simulink model "MagLev_1DOF_Slice_with_noise"  (R2020b)
settings: Solver=ode45  StartTime=0.0  StopTime=15  FixedStep=1e-5  RelTol=1e-3
values from neighbouring files (symbols this model uses):
  c = 0.005    [setup.m]
  caseNumber = 2    [setup.m]
  chi_0 = 0    [setup.m]
  dY_0 = 0.5    [setup.m]
  epsilon = 1e-3    (= 0.001)    [setup.m]
  eth10 = 0.0001    [setup.m]
  g = 9.81    [setup.m]
  gamma_ALCOS = 1000    [setup.m]
  gamma_s = 10    [setup.m]
  gamma_SLICE = 100    [setup.m]
  gamma_y = 10    [setup.m]
  k = 1    [setup.m]
  k0 = kk^3    (= 1000)    [setup.m]
  k1 = 3*kk^2    (= 300)    [setup.m]
  k2 = 3*kk    (= 30)    [setup.m]
  lambda_0 = -0.02    [setup.m]
  m = 0.0844    [setup.m]
  mu = 10    [setup.m]
  nu = 1    [setup.m]
  Omega = [ ... (first row only)    [setup.m]
  R = 2.52    [setup.m]
  s = [1; 2; 10; 20; 5; 7]    [setup.m]
  tt1 = 1    [setup.m]
  tt2 = 3    [setup.m]
  tt3 = 5    [setup.m]
  tt4 = 7    [setup.m]
  Y_0 = -1    [setup.m]
(part 2 of 2)

== matlab function MagLev_1DOF_Slice_with_noise/regression model/  regression model/terms of the real q4 ==
  data: q1 input; q2 input; phi1 input; phi2 input; psi input; omega1 input; omega2 input; W1 input size=10; W2 input size=6; W3 input size=2; k parameter; g parameter; m parameter; z output size=1; phi output size=6; w1 output size=10; w2 output size=6; lambda_0 parameter; w3 output; mu parameter
function [z, phi, w1, w2, w3] = fcn( q1, q2, phi1, phi2, psi, omega1, omega2, W1, W2, W3, k, g, m, lambda_0, mu)

theta = lambda_0;

psi1 = psi;
psi2 = psi1^2;

w1psi1 = W1(1);
w1psi2 = W1(2);
w1psi1w1psi1 = W1(3);
w1psi1w1psi2 = W1(4);
w1psi1w2psi1 = W1(5);
w1psi1w2psi2 = W1(6);
w1a1w1psi1 = W1(7);
w1a1w1psi2 = W1(8);
w1a1w2psi1 = W1(9);
w1a1w2psi2 = W1(10);

w2psi1 = W2(1);
w2psi2 = W2(2);
w2psi1w1psi1 = W2(3);
w2psi1w1psi2 = W2(4);
w2a1w1psi1 = W2(5);
w2a1w1psi2 = W2(6);

w3psi1 = W3(1);
w3psi2 = W3(2);

a1 = psi2 - 2*m*g*k;
psi1w1psi1 = psi1*w1psi1;
psi1w1psi2 = psi1*w1psi2;
psi1w2psi1 = psi1*w2psi1;
psi1w2psi2 = psi1*w2psi2;
a1w1psi1 = a1*w1psi1;
a1w1psi2 = a1*w1psi2;
a1w2psi1 = a1*w2psi1;
a1w2psi2 = a1*w2psi2;

w1 = [
  psi1;
  psi2;
  psi1w1psi1;
  psi1w1psi2;
  psi1w2psi1;
  psi1w2psi2;
  a1w1psi1;
  a1w1psi2;
  a1w2psi1;
  a1w2psi2
];

w2 = [
  psi1;
  psi2;
  psi1w1psi1;
  psi1w1psi2;
  a1w1psi1;
  a1w1psi2
];

w3 = [
  psi1;
  psi2;
];

% z = 2*k*mu*(k*m*q1*phi2 - q2*phi1) ...
%     + w2psi2*w1a1w1psi2 ...
%     - w1psi2*w1a1w2psi2 ...
%     - w1psi2*w2a1w1psi2;
% 
% phi1 =  ( omega1*w2psi2 - omega2*w1psi2 )*2*k^2*m*mu ...
%     - ( 2*w2psi1*w1a1w1psi2 + w2psi2*(2*w1psi1w1psi2 + 2*w1a1w1psi1) ) ...
%     + ( 2*w1psi1*w1a1w2psi2 + w1psi2*(2*w1psi1w2psi2 + 2*w1a1w2psi1) ) ...
%     + (2*w1psi1*w2a1w1psi2 + w1psi2*(2*w2psi1w1psi2 + 2*w2a1w1psi1));
%     
% phi2 = ( omega1*w2psi1 - omega2*w1psi1 )*4*k^2*m*mu ...
%     - ( w1a1w1psi2 + 4*w2psi1*(w1psi1w1psi2 + w1a1w1psi1) + w2psi2*(w1psi2 - 2*m*g*k + w2psi2 + 4*w1psi1w1psi1) ) ...
%     + ( w1a1w2psi2 + 4*w1psi1*(w1psi1w2psi2 + w1a1w2psi1) + w1psi2*(w1psi2 - 2*m*g*k + w3psi2 + 4*w1psi1w2psi1) ) ...
%     + (w2a1w1psi2 + 4*w1psi1*(w2psi1w1psi2 + w2a1w1psi1) + w1psi2*(w2psi2 - 2*m*g*k + w3psi2 + 4*w2psi1w1psi1));
% 
% phi3 = ( omega1 - omega2 )*2*k^2*m*mu ...
%     - ( 2*w1psi1w1psi2 + 2*w1a1w1psi1 + 2*w2psi1*(w1psi2 - 2*m*g*k + w2psi2 + 4*w1psi1w1psi1) + 2*w2psi2*(w1psi1 + w2psi1) ) ...
%     + ( 2*w1psi1w2psi2 + 2*w1a1w2psi1 + 2*w1psi1*(w1psi2 - 2*m*g*k + w3psi2 + 4*w1psi1w2psi1) + 2*w1psi2*(w1psi1 + w3psi1) ) ...
%     + (2*w2psi1w1psi2 + 2*w2a1w1psi1 + 2*w1psi1*(w2psi2 - 2*m*g*k + w3psi2 + 4*w2psi1w1psi1) + 2*w1psi2*(w2psi1 + w3psi1));
% 
% phi4 = - ( w1psi2 - 2*m*g*k + w2psi2 + 4*w1psi1w1psi1 + 4*w2psi1*(w1psi1 + w2psi1) + w2psi2 ) ...
%     + ( w1psi2 - 2*m*g*k + w3psi2 + 4*w1psi1w2psi1 + 4*w1psi1*(w1psi1 + w3psi1) + w1psi2 ) ...
%     + (w2psi2 - 2*m*g*k + w3psi2 + 4*w2psi1w1psi1 + 4*w1psi1*(w2psi1 + w3psi1) + w1psi2);

z = 2*k*mu*(k*m*q1*phi2 - q2*phi1) ...
    - w1psi2*(w1a1w2psi2 + w2a1w1psi2) ...
    + w2psi2*w1a1w1psi2;

phi1 =  ( omega1*w2psi2 - omega2*w1psi2 )*2*k^2*m*mu ...
    + 2*w1psi1*(w1a1w2psi2 + w2a1w1psi2) ...
    + 2*w1psi2*(w1psi1w2psi2 + w1a1w2psi1 + w2psi1w1psi2 + w2a1w1psi1) ...
    - 2*w2psi1*w1a1w1psi2 ...
    - 2*w2psi2*(w1psi1w1psi2 + w1a1w1psi1);
    
phi2 = ( omega1*w2psi1 - omega2*w1psi1 )*4*k^2*m*mu ...
    + 2*m*g*k*(w2psi2 - 2*w1psi2) ...
    + (w1psi2)^2 - (w2psi2)^2 ...
    + 4*w1psi1*(w1psi1w2psi2 + w1a1w2psi1 + w2psi1w1psi2 + w2a1w1psi1) ...
    + 2*w1psi2*(w3psi2 + 2*w1psi1w2psi1 + 2*w2psi1w1psi1) ...
    - 4*w2psi1*(w1psi1w1psi2 + w1a1w1psi1) ...
    - w1a1w1psi2 + w1a1w2psi2 ...
    + w2a1w1psi2 ...
    - 4*w2psi2*w1psi1w1psi1;

phi3 = ( omega1 - omega2 )*2*k^2*m*mu ...
    + 4*m*g*k*(w2psi1 - 2*w1psi1)  ...
    + 4*w1psi1*(w1psi2 + w3psi2 + 2*w1psi1w2psi1 + 2*w2psi1w1psi1) ...
    + 4*w1psi2*w3psi1 ...
    - 4*w2psi1*( w2psi2 + 2*w1psi1w1psi1) ...
    - 2*w1psi1w1psi2 + 2*w1psi1w2psi2+ 2*w2psi1w1psi2 ...
    - 2*w1a1w1psi1+ 2*w1a1w2psi1 + 2*w2a1w1psi1;

phi4 = - 2*m*g*k + 2*w1psi2 - w2psi2 + 2*w3psi2 - 4*w2psi1*w2psi1 ...
    + 4*w1psi1*w1psi1 + 8*w1psi1*w3psi1 ...
    - 4*w1psi1w1psi1 + 4*w1psi1w2psi1 ...
    + 4*w2psi1w1psi1;

phi5 = - 2*w2psi1 + 4*w3psi1 + 4*w1psi1;

phi6 = 1;

phi = [
    phi1;
    phi2;
    phi3;
    phi4;
    phi5;
    phi6
];

== matlab function MagLev_1DOF_Slice_with_noise/Controller ==
  data: Yd input size=4; u output size=1; X input size=3; c parameter; k parameter; R parameter; g parameter; m parameter; k0 parameter; k1 parameter; k2 parameter
function u = fcn(Yd, X, c, k, R, g, m, k0, k1, k2)

Y = X(1);
dY = X(2)/m;
lambda = X(3);

F = 0.5*lambda^2/k;

v = Yd(4) - k2*( (F/m - g) - Yd(3) ) - k1*( dY - Yd(2) ) - k0*( Y - Yd(1));

u = sqrt(0.5*k/F)*m*v + R*(c - Y)*sqrt(2*F/k);

== matlab function MagLev_1DOF_Slice_with_noise/Controller1 ==
  data: Yd input size=4; u output size=1; X input size=3; c parameter; k parameter; R parameter; g parameter; m parameter; k0 parameter; k1 parameter; k2 parameter
function u = fcn(Yd, X, c, k, R, g, m, k0, k1, k2)

Y = X(1);
dY = X(2)/m;
lambda = X(3);

F = 0.5*lambda^2/k;

v = Yd(4) - k2*( (F/m - g) - Yd(3) ) - k1*( dY - Yd(2) ) - k0*( Y - Yd(1));

u = sqrt(0.5*k/F)*m*v + R*(c - Y)*sqrt(2*F/k);

== matlab function MagLev_1DOF_Slice_with_noise/regression model/Vectorize/q1/terms of the q1 est ==
  data: y input; u input; psi input; omega1 input; R parameter; term1 output; term2 output; term3 output
function [term1, term2, term3] = fcn( y, u, psi, omega1, R )

term1 = y*(u - R*y);
term2 = psi*omega1;
term3 = (u - R*y)*omega1;

== matlab function MagLev_1DOF_Slice_with_noise/Estimation ALCOS/DREM2 ==
  data: in1 input size=6; newreg output; in2 input size=6 =in2; y1 output; y2 output; y3 output; y4 output; in3 input size=6; in4 input size=6; in5 input size=6; y5 output
function [newreg,y1,y2,y3,y4,y5] = fcn(in1,in2,in3,in4,in5)


a11=in1(1); a12=in1(2); a13=in1(3); a14=in1(4); a15=in1(5);

a21=in2(1); a22=in2(2); a23=in2(3); a24=in2(4); a25=in2(5);

a31=in3(1); a32=in3(2); a33=in3(3); a34=in3(4); a35=in3(5);

a41=in4(1); a42=in4(2); a43=in4(3); a44=in4(4); a45=in4(5);

a51=in5(1); a52=in5(2); a53=in5(3); a54=in5(4); a55=in5(5);

RegM=[a11  a12  a13  a14  a15; a21  a22  a23  a24  a25; a31  a32  a33  a34  a35; a41  a42  a43  a44  a45; a51  a52  a53  a54  a55];

newreg=det(RegM);

adj1=[a22*a33*a44*a55 - a22*a33*a45*a54 - a22*a34*a43*a55 + a22*a34*a45*a53 + a22*a35*a43*a54 - a22*a35*a44*a53 - a23*a32*a44*a55 + a23*a32*a45*a54 ...
+ a23*a34*a42*a55 - a23*a34*a45*a52 - a23*a35*a42*a54 + a23*a35*a44*a52 + a24*a32*a43*a55 - a24*a32*a45*a53 - a24*a33*a42*a55 + a24*a33*a45*a52 ...
+ a24*a35*a42*a53 - a24*a35*a43*a52 - a25*a32*a43*a54 + a25*a32*a44*a53 + a25*a33*a42*a54 - a25*a33*a44*a52 - a25*a34*a42*a53 + a25*a34*a43*a52, 
a12*a33*a45*a54 - a12*a33*a44*a55 + a12*a34*a43*a55 - a12*a34*a45*a53 - a12*a35*a43*a54 + a12*a35*a44*a53 + a13*a32*a44*a55 - a13*a32*a45*a54 - ...
a13*a34*a42*a55 + a13*a34*a45*a52 + a13*a35*a42*a54 - a13*a35*a44*a52 - a14*a32*a43*a55 + a14*a32*a45*a53 + a14*a33*a42*a55 - a14*a33*a45*a52 - ...
a14*a35*a42*a53 + a14*a35*a43*a52 + a15*a32*a43*a54 - a15*a32*a44*a53 - a15*a33*a42*a54 + a15*a33*a44*a52 + a15*a34*a42*a53 - a15*a34*a43*a52, 
a12*a23*a44*a55 - a12*a23*a45*a54 - a12*a24*a43*a55 + a12*a24*a45*a53 + a12*a25*a43*a54 - a12*a25*a44*a53 - a13*a22*a44*a55 + a13*a22*a45*a54 ...
+ a13*a24*a42*a55 - a13*a24*a45*a52 - a13*a25*a42*a54 + a13*a25*a44*a52 + a14*a22*a43*a55 - a14*a22*a45*a53 - a14*a23*a42*a55 + a14*a23*a45*a52 ...
+ a14*a25*a42*a53 - a14*a25*a43*a52 - a15*a22*a43*a54 + a15*a22*a44*a53 + a15*a23*a42*a54 - a15*a23*a44*a52 - a15*a24*a42*a53 + a15*a24*a43*a52, 
a12*a23*a35*a54 - a12*a23*a34*a55 + a12*a24*a33*a55 - a12*a24*a35*a53 - a12*a25*a33*a54 + a12*a25*a34*a53 + a13*a22*a34*a55 - a13*a22*a35*a54 ...
- a13*a24*a32*a55 + a13*a24*a35*a52 + a13*a25*a32*a54 - a13*a25*a34*a52 - a14*a22*a33*a55 + a14*a22*a35*a53 + a14*a23*a32*a55 - a14*a23*a35*a52 ...
- a14*a25*a32*a53 + a14*a25*a33*a52 + a15*a22*a33*a54 - a15*a22*a34*a53 - a15*a23*a32*a54 + a15*a23*a34*a52 + a15*a24*a32*a53 - a15*a24*a33*a52, 
a12*a23*a34*a45 - a12*a23*a35*a44 - a12*a24*a33*a45 + a12*a24*a35*a43 + a12*a25*a33*a44 - a12*a25*a34*a43 - a13*a22*a34*a45 + a13*a22*a35*a44 ...
+ a13*a24*a32*a45 - a13*a24*a35*a42 - a13*a25*a32*a44 + a13*a25*a34*a42 + a14*a22*a33*a45 - a14*a22*a35*a43 - a14*a23*a32*a45 + a14*a23*a35*a42 ...
+ a14*a25*a32*a43 - a14*a25*a33*a42 - a15*a22*a33*a44 + a15*a22*a34*a43 + a15*a23*a32*a44 - a15*a23*a34*a42 - a15*a24*a32*a43 + a15*a24*a33*a42];

adj2=[a21*a33*a45*a54 - a21*a33*a44*a55 + a21*a34*a43*a55 - a21*a34*a45*a53 - a21*a35*a43*a54 + a21*a35*a44*a53 + a23*a31*a44*a55 - a23*a31*a45*a54 ...
- a23*a34*a41*a55 + a23*a34*a45*a51 + a23*a35*a41*a54 - a23*a35*a44*a51 - a24*a31*a43*a55 + a24*a31*a45*a53 + a24*a33*a41*a55 - a24*a33*a45*a51 ...
- a24*a35*a41*a53 + a24*a35*a43*a51 + a25*a31*a43*a54 - a25*a31*a44*a53 - a25*a33*a41*a54 + a25*a33*a44*a51 + a25*a34*a41*a53 - a25*a34*a43*a51, 
a11*a33*a44*a55 - a11*a33*a45*a54 - a11*a34*a43*a55 + a11*a34*a45*a53 + a11*a35*a43*a54 - a11*a35*a44*a53 - a13*a31*a44*a55 + a13*a31*a45*a54 ...
+ a13*a34*a41*a55 - a13*a34*a45*a51 - a13*a35*a41*a54 + a13*a35*a44*a51 + a14*a31*a43*a55 - a14*a31*a45*a53 - a14*a33*a41*a55 + a14*a33*a45*a51 ...
+ a14*a35*a41*a53 - a14*a35*a43*a51 - a15*a31*a43*a54 + a15*a31*a44*a53 + a15*a33*a41*a54 - a15*a33*a44*a51 - a15*a34*a41*a53 + a15*a34*a43*a51, 
a11*a23*a45*a54 - a11*a23*a44*a55 + a11*a24*a43*a55 - a11*a24*a45*a53 - a11*a25*a43*a54 + a11*a25*a44*a53 + a13*a21*a44*a55 - a13*a21*a45*a54 ...
- a13*a24*a41*a55 + a13*a24*a45*a51 + a13*a25*a41*a54 - a13*a25*a44*a51 - a14*a21*a43*a55 + a14*a21*a45*a53 + a14*a23*a41*a55 - a14*a23*a45*a51...
- a14*a25*a41*a53 + a14*a25*a43*a51 + a15*a21*a43*a54 - a15*a21*a44*a53 - a15*a23*a41*a54 + a15*a23*a44*a51 + a15*a24*a41*a53 - a15*a24*a43*a51, 
a11*a23*a34*a55 - a11*a23*a35*a54 - a11*a24*a33*a55 + a11*a24*a35*a53 + a11*a25*a33*a54 - a11*a25*a34*a53 - a13*a21*a34*a55 + a13*a21*a35*a54 ...
+ a13*a24*a31*a55 - a13*a24*a35*a51 - a13*a25*a31*a54 + a13*a25*a34*a51 + a14*a21*a33*a55 - a14*a21*a35*a53 - a14*a23*a31*a55 + a14*a23*a35*a51 ...
+ a14*a25*a31*a53 - a14*a25*a33*a51 - a15*a21*a33*a54 + a15*a21*a34*a53 + a15*a23*a31*a54 - a15*a23*a34*a51 - a15*a24*a31*a53 + a15*a24*a33*a51, 
a11*a23*a35*a44 - a11*a23*a34*a45 + a11*a24*a33*a45 - a11*a24*a35*a43 - a11*a25*a33*a44 + a11*a25*a34*a43 + a13*a21*a34*a45 - a13*a21*a35*a44...
- a13*a24*a31*a45 + a13*a24*a35*a41 + a13*a25*a31*a44 - a13*a25*a34*a41 - a14*a21*a33*a45 + a14*a21*a35*a43 + a14*a23*a31*a45 - a14*a23*a35*a41 ...
- a14*a25*a31*a43 + a14*a25*a33*a41 + a15*a21*a33*a44 - a15*a21*a34*a43 - a15*a23*a31*a44 + a15*a23*a34*a41 + a15*a24*a31*a43 - a15*a24*a33*a41];

adj3=[a21*a32*a44*a55 - a21*a32*a45*a54 - a21*a34*a42*a55 + a21*a34*a45*a52 + a21*a35*a42*a54 - a21*a35*a44*a52 - a22*a31*a44*a55 + a22*a31*a45*a54 ...
+ a22*a34*a41*a55 - a22*a34*a45*a51 - a22*a35*a41*a54 + a22*a35*a44*a51 + a24*a31*a42*a55 - a24*a31*a45*a52 - a24*a32*a41*a55 + a24*a32*a45*a51...
+ a24*a35*a41*a52 - a24*a35*a42*a51 - a25*a31*a42*a54 + a25*a31*a44*a52 + a25*a32*a41*a54 - a25*a32*a44*a51 - a25*a34*a41*a52 + a25*a34*a42*a51, 
a11*a32*a45*a54 - a11*a32*a44*a55 + a11*a34*a42*a55 - a11*a34*a45*a52 - a11*a35*a42*a54 + a11*a35*a44*a52 + a12*a31*a44*a55 - a12*a31*a45*a54 ...
- a12*a34*a41*a55 + a12*a34*a45*a51 + a12*a35*a41*a54 - a12*a35*a44*a51 - a14*a31*a42*a55 + a14*a31*a45*a52 + a14*a32*a41*a55 - a14*a32*a45*a51 ...
- a14*a35*a41*a52 + a14*a35*a42*a51 + a15*a31*a42*a54 - a15*a31*a44*a52 - a15*a32*a41*a54 + a15*a32*a44*a51 + a15*a34*a41*a52 - a15*a34*a42*a51, 
a11*a22*a44*a55 - a11*a22*a45*a54 - a11*a24*a42*a55 + a11*a24*a45*a52 + a11*a25*a42*a54 - a11*a25*a44*a52 - a12*a21*a44*a55 + a12*a21*a45*a54 ...
+ a12*a24*a41*a55 - a12*a24*a45*a51 - a12*a25*a41*a54 + a12*a25*a44*a51 + a14*a21*a42*a55 - a14*a21*a45*a52 - a14*a22*a41*a55 + a14*a22*a45*a51 ...
+ a14*a25*a41*a52 - a14*a25*a42*a51 - a15*a21*a42*a54 + a15*a21*a44*a52 + a15*a22*a41*a54 - a15*a22*a44*a51 - a15*a24*a41*a52 + a15*a24*a42*a51, 
a11*a22*a35*a54 - a11*a22*a34*a55 + a11*a24*a32*a55 - a11*a24*a35*a52 - a11*a25*a32*a54 + a11*a25*a34*a52 + a12*a21*a34*a55 - a12*a21*a35*a54...
- a12*a24*a31*a55 + a12*a24*a35*a51 + a12*a25*a31*a54 - a12*a25*a34*a51 - a14*a21*a32*a55 + a14*a21*a35*a52 + a14*a22*a31*a55 - a14*a22*a35*a51 ...
- a14*a25*a31*a52 + a14*a25*a32*a51 + a15*a21*a32*a54 - a15*a21*a34*a52 - a15*a22*a31*a54 + a15*a22*a34*a51 + a15*a24*a31*a52 - a15*a24*a32*a51, 
a11*a22*a34*a45 - a11*a22*a35*a44 - a11*a24*a32*a45 + a11*a24*a35*a42 + a11*a25*a32*a44 - a11*a25*a34*a42 - a12*a21*a34*a45 + a12*a21*a35*a44 ...
+ a12*a24*a31*a45 - a12*a24*a35*a41 - a12*a25*a31*a44 + a12*a25*a34*a41 + a14*a21*a32*a45 - a14*a21*a35*a42 - a14*a22*a31*a45 + a14*a22*a35*a41 ...
+ a14*a25*a31*a42 - a14*a25*a32*a41 - a15*a21*a32*a44 + a15*a21*a34*a42 + a15*a22*a31*a44 - a15*a22*a34*a41 - a15*a24*a31*a42 + a15*a24*a32*a41];

adj4=[a21*a32*a45*a53 - a21*a32*a43*a55 + a21*a33*a42*a55 - a21*a33*a45*a52 - a21*a35*a42*a53 + a21*a35*a43*a52 + a22*a31*a43*a55 - a22*a31*a45*a53 ...
- a22*a33*a41*a55 + a22*a33*a45*a51 + a22*a35*a41*a53 - a22*a35*a43*a51 - a23*a31*a42*a55 + a23*a31*a45*a52 + a23*a32*a41*a55 - a23*a32*a45*a51 ...
- a23*a35*a41*a52 + a23*a35*a42*a51 + a25*a31*a42*a53 - a25*a31*a43*a52 - a25*a32*a41*a53 + a25*a32*a43*a51 + a25*a33*a41*a52 - a25*a33*a42*a51, 
a11*a32*a43*a55 - a11*a32*a45*a53 - a11*a33*a42*a55 + a11*a33*a45*a52 + a11*a35*a42*a53 - a11*a35*a43*a52 - a12*a31*a43*a55 + a12*a31*a45*a53 ...
+ a12*a33*a41*a55 - a12*a33*a45*a51 - a12*a35*a41*a53 + a12*a35*a43*a51 + a13*a31*a42*a55 - a13*a31*a45*a52 - a13*a32*a41*a55 + a13*a32*a45*a51 ...
+ a13*a35*a41*a52 - a13*a35*a42*a51 - a15*a31*a42*a53 + a15*a31*a43*a52 + a15*a32*a41*a53 - a15*a32*a43*a51 - a15*a33*a41*a52 + a15*a33*a42*a51, 
a11*a22*a45*a53 - a11*a22*a43*a55 + a11*a23*a42*a55 - a11*a23*a45*a52 - a11*a25*a42*a53 + a11*a25*a43*a52 + a12*a21*a43*a55 - a12*a21*a45*a53 ...
- a12*a23*a41*a55 + a12*a23*a45*a51 + a12*a25*a41*a53 - a12*a25*a43*a51 - a13*a21*a42*a55 + a13*a21*a45*a52 + a13*a22*a41*a55 - a13*a22*a45*a51...
- a13*a25*a41*a52 + a13*a25*a42*a51 + a15*a21*a42*a53 - a15*a21*a43*a52 - a15*a22*a41*a53 + a15*a22*a43*a51 + a15*a23*a41*a52 - a15*a23*a42*a51, 
a11*a22*a33*a55 - a11*a22*a35*a53 - a11*a23*a32*a55 + a11*a23*a35*a52 + a11*a25*a32*a53 - a11*a25*a33*a52 - a12*a21*a33*a55 + a12*a21*a35*a53 ...
+ a12*a23*a31*a55 - a12*a23*a35*a51 - a12*a25*a31*a53 + a12*a25*a33*a51 + a13*a21*a32*a55 - a13*a21*a35*a52 - a13*a22*a31*a55 + a13*a22*a35*a51 ...
+ a13*a25*a31*a52 - a13*a25*a32*a51 - a15*a21*a32*a53 + a15*a21*a33*a52 + a15*a22*a31*a53 - a15*a22*a33*a51 - a15*a23*a31*a52 + a15*a23*a32*a51,
a11*a22*a35*a43 - a11*a22*a33*a45 + a11*a23*a32*a45 - a11*a23*a35*a42 - a11*a25*a32*a43 + a11*a25*a33*a42 + a12*a21*a33*a45 - a12*a21*a35*a43 ...
- a12*a23*a31*a45 + a12*a23*a35*a41 + a12*a25*a31*a43 - a12*a25*a33*a41 - a13*a21*a32*a45 + a13*a21*a35*a42 + a13*a22*a31*a45 - a13*a22*a35*a41 ...
- a13*a25*a31*a42 + a13*a25*a32*a41 + a15*a21*a32*a43 - a15*a21*a33*a42 - a15*a22*a31*a43 + a15*a22*a33*a41 + a15*a23*a31*a42 - a15*a23*a32*a41];

adj5=[a21*a32*a43*a54 - a21*a32*a44*a53 - a21*a33*a42*a54 + a21*a33*a44*a52 + a21*a34*a42*a53 - a21*a34*a43*a52 - a22*a31*a43*a54 + a22*a31*a44*a53...
+ a22*a33*a41*a54 - a22*a33*a44*a51 - a22*a34*a41*a53 + a22*a34*a43*a51 + a23*a31*a42*a54 - a23*a31*a44*a52 - a23*a32*a41*a54 + a23*a32*a44*a51 ...
+ a23*a34*a41*a52 - a23*a34*a42*a51 - a24*a31*a42*a53 + a24*a31*a43*a52 + a24*a32*a41*a53 - a24*a32*a43*a51 - a24*a33*a41*a52 + a24*a33*a42*a51, 
a11*a32*a44*a53 - a11*a32*a43*a54 + a11*a33*a42*a54 - a11*a33*a44*a52 - a11*a34*a42*a53 + a11*a34*a43*a52 + a12*a31*a43*a54 - a12*a31*a44*a53 ...
- a12*a33*a41*a54 + a12*a33*a44*a51 + a12*a34*a41*a53 - a12*a34*a43*a51 - a13*a31*a42*a54 + a13*a31*a44*a52 + a13*a32*a41*a54 - a13*a32*a44*a51 ...
- a13*a34*a41*a52 + a13*a34*a42*a51 + a14*a31*a42*a53 - a14*a31*a43*a52 - a14*a32*a41*a53 + a14*a32*a43*a51 + a14*a33*a41*a52 - a14*a33*a42*a51,
a11*a22*a43*a54 - a11*a22*a44*a53 - a11*a23*a42*a54 + a11*a23*a44*a52 + a11*a24*a42*a53 - a11*a24*a43*a52 - a12*a21*a43*a54 + a12*a21*a44*a53 ...
+ a12*a23*a41*a54 - a12*a23*a44*a51 - a12*a24*a41*a53 + a12*a24*a43*a51 + a13*a21*a42*a54 - a13*a21*a44*a52 - a13*a22*a41*a54 + a13*a22*a44*a51...
+ a13*a24*a41*a52 - a13*a24*a42*a51 - a14*a21*a42*a53 + a14*a21*a43*a52 + a14*a22*a41*a53 - a14*a22*a43*a51 - a14*a23*a41*a52 + a14*a23*a42*a51,
a11*a22*a34*a53 - a11*a22*a33*a54 + a11*a23*a32*a54 - a11*a23*a34*a52 - a11*a24*a32*a53 + a11*a24*a33*a52 + a12*a21*a33*a54 - a12*a21*a34*a53 ...
- a12*a23*a31*a54 + a12*a23*a34*a51 + a12*a24*a31*a53 - a12*a24*a33*a51 - a13*a21*a32*a54 + a13*a21*a34*a52 + a13*a22*a31*a54 - a13*a22*a34*a51 ...
- a13*a24*a31*a52 + a13*a24*a32*a51 + a14*a21*a32*a53 - a14*a21*a33*a52 - a14*a22*a31*a53 + a14*a22*a33*a51 + a14*a23*a31*a52 - a14*a23*a32*a51,
a11*a22*a33*a44 - a11*a22*a34*a43 - a11*a23*a32*a44 + a11*a23*a34*a42 + a11*a24*a32*a43 - a11*a24*a33*a42 - a12*a21*a33*a44 + a12*a21*a34*a43 ...
+ a12*a23*a31*a44 - a12*a23*a34*a41 - a12*a24*a31*a43 + a12*a24*a33*a41 + a13*a21*a32*a44 - a13*a21*a34*a42 - a13*a22*a31*a44 + a13*a22*a34*a41 ...
+ a13*a24*a31*a42 - a13*a24*a32*a41 - a14*a21*a32*a43 + a14*a21*a33*a42 + a14*a22*a31*a43 - a14*a22*a33*a41 - a14*a23*a31*a42 + a14*a23*a32*a41];



y1 = adj1'*[in1(6);in2(6);in3(6);in4(6);in5(6)];
y2 = adj2'*[in1(6);in2(6);in3(6);in4(6);in5(6)];
y3 = adj3'*[in1(6);in2(6);in3(6);in4(6);in5(6)];
y4 = adj4'*[in1(6);in2(6);in3(6);in4(6);in5(6)];
y5 = adj5'*[in1(6);in2(6);in3(6);in4(6);in5(6)];
